simulink model "nonlinear_closed"  (R2024a)
settings: Solver=VariableStepAuto  StartTime=0.0  StopTime=5  MaxStep=1e-4  RelTol=1e-4
values from neighbouring files (symbols this model uses):
  beta = m * lc    (= 40.0551)    [t_411.m]    (also in t_412.m; t_413.m; t_414.m; t_42.m)
  f = 0    [t_411.m]    (also in t_412.m; t_413.m; t_414.m; t_42.m)
  g = 9.81    [t_411.m]    (also in t_412.m; t_413.m; t_414.m; t_42.m)
  J = (1/3)*m1*l^2 + m2*l^2    (= 62.720658)    [t_411.m]    (also in t_412.m; t_413.m; t_414.m; t_42.m)
  K = -Y * inv(P)    [t_411.m]    (also in t_412.m; t_413.m; t_414.m; t_42.m = 1.0e+05 *[-0.7358   -0.5165   -2.4382   -0.9334])
  M = 658.36    [t_411.m]    (also in t_412.m; t_413.m; t_414.m; t_42.m)
  m = m1 + m2    (= 30.46)    [t_411.m]    (also in t_412.m; t_413.m; t_414.m; t_42.m)
  x0 = x0_list{i}    [t_411.m]    (also in t_412.m = [0.1; 0.2; 0.03; 0.12]; t_413.m; t_414.m = [0.1; 0.2; 0.03; 0.12]; t_42.m = [0.1; 0.2; 0.03; 0.12])
settings Model: Creator=eva  LastModifiedBy=eva

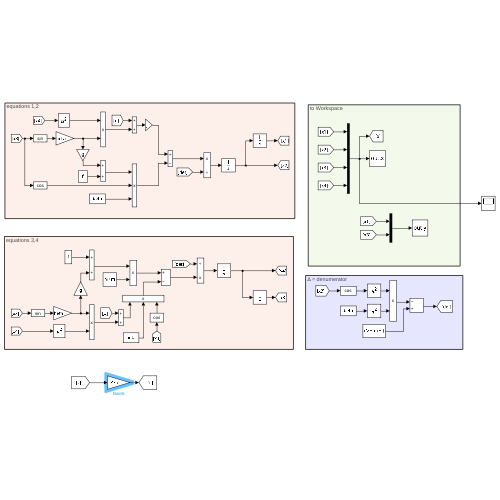
[thumbnail: Simulink's stored preview of the top-level diagram]
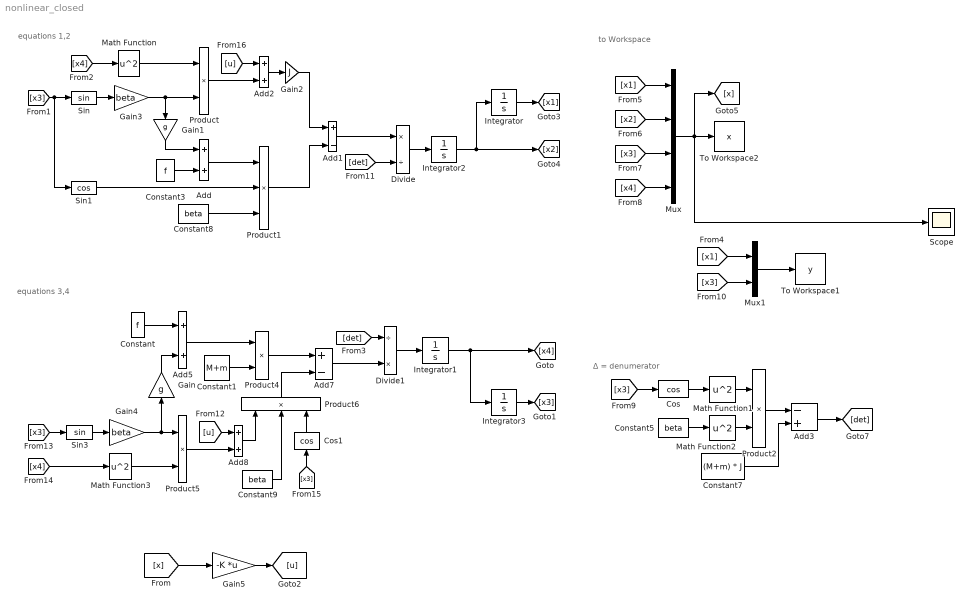
== system nonlinear_closed ==
  note: equations 3,4
  note: Δ = denumerator
  note: to Workspace
  note: equations 1,2
  Add{,2,5,8} (4 alike) : Sum
  Add1 : Sum  Inputs=+-
  Add3 : Sum  Inputs=-+
  Add7 : Sum  Inputs=+-
  Constant : Constant  Value=f
  Constant1 : Constant  Value=M+m
  Constant3 : Constant  Value=f
  Constant5 : Constant  Value=beta
  Constant7 : Constant  Value=(M+m) * J
  Constant8 : Constant  Value=beta
  Constant9 : Constant  Value=beta
  Cos : Trigonometry  Operator=cos
  Cos1 : Trigonometry  Operator=cos
  Divide : Product  Inputs=*/
  Divide1 : Product  Inputs=/*
  Gain : Gain  Gain=g
  Gain1 : Gain  Gain=g
  Gain2 : Gain  Gain=J
  Gain3 : Gain  Gain=beta
  Gain4 : Gain  Gain=beta
  Gain5 : Gain  Gain=-K  Multiplication=Matrix(K*u)
  Integrator : Integrator  InitialCondition=x0(1)
  Integrator1 : Integrator  InitialCondition=x0(4)
  Integrator2 : Integrator  InitialCondition=x0(2)
  Integrator3 : Integrator  InitialCondition=x0(3)
  Math Function{,1..3} (4 alike) : Math  Operator=square
  Mux : Mux
  Mux1 : Mux  Inputs=2
  Product{,2,4..5} (4 alike) : Product
  Product1 : Product  Inputs=3
  Product6 : Product  Inputs=3
  Scope : Scope
  Sin : Trigonometry
  Sin1 : Trigonometry  Operator=cos
  Sin3 : Trigonometry
  To Workspace1 : ToWorkspace  VariableName=y  SaveFormat=Structure With Time  SampleTime=-1
  To Workspace2 : ToWorkspace  VariableName=x  SaveFormat=Structure With Time  SampleTime=-1
  wires:
  Product/1 -> Add2/2
  [x4] -> Mux/4
  Integrator3/1 -> [x3]
  Integrator2/1 -> [x2], Integrator/1
  [det] -> Divide/2
  Divide1/1 -> Integrator1/1
  Constant9/1 -> Product6/2
  Mux1/1 -> To Workspace1/1
  [u] -> Add8/1
  [x1] -> Mux/1
  Add/1 -> Product1/1
  Add8/1 -> Product6/1
  [x4] -> Math Function3/1
  Integrator1/1 -> [x4], Integrator3/1
  [x3] -> Mux1/2
  Product2/1 -> Add3/1
  [x3] -> Sin/1, Sin1/1
  Constant3/1 -> Add/2
  Constant1/1 -> Product4/2
  Cos/1 -> Math Function1/1
  Sin1/1 -> Product1/2
  Sin/1 -> Gain3/1
  Constant5/1 -> Math Function2/1
  [x4] -> Math Function/1
  Constant8/1 -> Product1/3
  Gain2/1 -> Add1/1
  Mux/1 -> [x], Scope/1, To Workspace2/1
  Add7/1 -> Divide1/2
  Add2/1 -> Gain2/1
  Constant/1 -> Add5/1
  Cos1/1 -> Product6/3
  Product4/1 -> Add7/1
  Product1/1 -> Add1/2
  Gain3/1 -> Product/2, Gain1/1
  Gain/1 -> Add5/2
  [x3] -> Cos/1
  Product5/1 -> Add8/2
  [x3] -> Mux/3
  Constant7/1 -> Add3/2
  Product6/1 -> Add7/2
  [x2] -> Mux/2
  Add1/1 -> Divide/1
  [x3] -> Cos1/1
  [det] -> Divide1/1
  Integrator/1 -> [x1]
  Math Function2/1 -> Product2/2
  Add3/1 -> [det]
  Math Function1/1 -> Product2/1
  [x1] -> Mux1/1
  Math Function3/1 -> Product5/2
  Math Function/1 -> Product/1
  [x3] -> Sin3/1
  Divide/1 -> Integrator2/1
  Gain4/1 -> Product5/1, Gain/1
  Gain1/1 -> Add/1
  Add5/1 -> Product4/1
  Sin3/1 -> Gain4/1
  [x] -> Gain5/1
  Gain5/1 -> [u]
  [u] -> Add2/1
